simulink model "encoder2"  (R2022a)
settings: Solver=VariableStepAuto  StartTime=0.0  StopTime=10.0  RelTol=1e-3
libraries: simulink x3, spsSampleandHoldLib x1
settings Model: Creator=mluser  LastModifiedBy=mluser
settings ModelReferenceCC: EnableRefExpFcnMdlSchedulingChecks=off
settings RTWCC: Description=Generic Real-Time Target

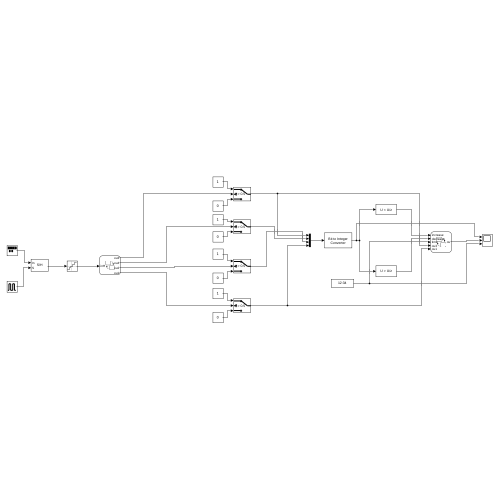
[thumbnail: Simulink's stored preview of the top-level diagram]
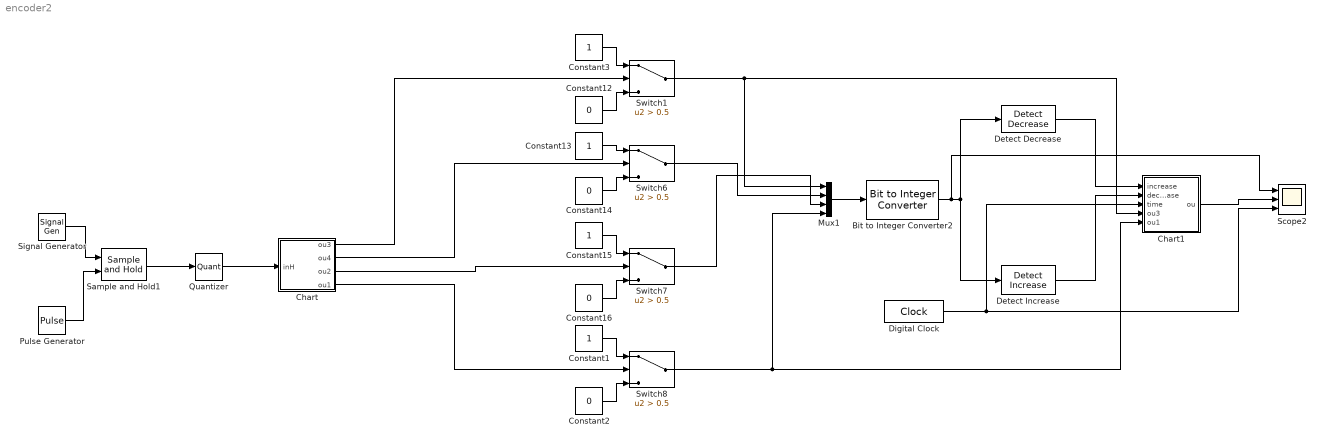
== system encoder2 ==
  Bit to Integer Converter2 : simulink/Logic and Bit Operations/Bit to Integer Converter  nbits=4  bitOrder=MSB first  signedOutputValues=Unsigned  outDtype=Inherit via internal rule  outDtypeSigned=Inherit via internal rule
  Chart : Stateflow chart  TreatAsAtomicUnit=on
  Chart1 : Stateflow chart  TreatAsAtomicUnit=on
  Constant{1,3,13,15} (4 alike) : Constant
  Constant{2,12,14,16} (4 alike) : Constant  Value=0
  Detect Decrease : simulink/Logic and Bit Operations/Detect Decrease  vinit=0.0  OutDataTypeStr=boolean
  Detect Increase : simulink/Logic and Bit Operations/Detect Increase  vinit=0.0  OutDataTypeStr=boolean
  Digital Clock : DigitalClock  SampleTime=0.1
  Mux1 : Mux
  Pulse Generator : DiscretePulseGenerator  PulseType=Time based  Period=0.1  PulseWidth=5
  Quantizer : Quantizer
  Sample and Hold1 : spsSampleandHoldLib/Sample and Hold  ic=0  Ts=0.1
  Scope2 : Scope  NumInputPorts=3
  Signal Generator : SignalGenerator  Amplitude=40  Units=rad/sec
  Switch{1,6..8} (4 alike) : Switch  Criteria=u2 > Threshold  Threshold=0.5  SaturateOnIntegerOverflow=off  InputSameDT=off
  wires:
  Pulse Generator/1 -> Sample and Hold1/2
  Signal Generator/1 -> Sample and Hold1/1
  Sample and Hold1/1 -> Quantizer/1
  Quantizer/1 -> Chart/1(inH)
  Constant3/1 -> Switch1/1
  Constant14/1 -> Switch6/3
  Chart/2(ou4) -> Switch6/2
  Switch7/1 -> Mux1/3
  Constant15/1 -> Switch7/1
  Constant13/1 -> Switch6/1
  Switch6/1 -> Mux1/2
  Chart/1(ou3) -> Switch1/2
  Constant16/1 -> Switch7/3
  Chart/3(ou2) -> Switch7/2
  Constant12/1 -> Switch1/3
  Switch1/1 -> Chart1/4(ou3), Mux1/1
  Constant1/1 -> Switch8/1
  Constant2/1 -> Switch8/3
  Chart/4(ou1) -> Switch8/2
  Switch8/1 -> Chart1/5(ou1), Mux1/4
  Mux1/1 -> Bit to Integer Converter2/1
  Bit to Integer Converter2/1 -> Scope2/1, Detect Decrease/1, Detect Increase/1
  Detect Decrease/1 -> Chart1/1(increase)
  Detect Increase/1 -> Chart1/2(decrease)
  Chart1/1(ou) -> Scope2/2
  Digital Clock/1 -> Scope2/3, Chart1/3(time)

== stateflow chart encoder2/Chart ==
  (default) -> (junction 3) : {ou1=0;
      | ou2=0;
      | ou3=0;
      | ou4=0;
      | }
  (junction 3) -> (junction 28) [order 2] : [inH==0]
  (junction 28) -> (junction 44) : {ou1=0;ou2=0;ou3=0;ou4=0;}
  (junction 3) -> (junction 10) [order 1]
  (junction 44) -> (junction 43)
  (junction 10) -> (junction 8) [order 1] : [inH<=10]
  (junction 8) -> (junction 43) : {ou1=1;ou2=0;ou3=0;ou4=0;}
  (junction 10) -> (junction 12) [order 2]
  (junction 43) -> (junction 42)
  (junction 16) -> (junction 42) : {ou1=1;ou2=1;ou3=0;ou4=0;}
  (junction 12) -> (junction 16) [order 1] : [inH>10&&inH<=20]
  (junction 42) -> (junction 41)
  (junction 12) -> (junction 19) [order 2]
  (junction 19) -> (junction 18) [order 1] : [inH>20&&inH<=30]
  (junction 18) -> (junction 41) : {ou1=1;ou2=1;ou3=1;ou4=0;}
  (junction 41) -> (junction 63)
  (junction 19) -> (junction 61) [order 2]
  (junction 61) -> (junction 62) : [inH>30]
  (junction 62) -> (junction 63) : {ou1=1;ou2=1;ou3=1;ou4=1;}
  data: ou3 output; ou4 output; ou2 output; ou1 output; inH input

== stateflow chart encoder2/Chart1 ==
  (default) -> (junction 3)
  (junction 3) -> (junction 28) [order 2] : [increase==1&&time>0]
  (junction 28) -> (junction 44) : {ou=1;}
  (junction 3) -> (junction 10) [order 1]
  (junction 44) -> (junction 43)
  (junction 10) -> (junction 8) [order 1] : [decrease==1&&time>0]
  (junction 8) -> (junction 43) : {ou=0;}
  (junction 10) -> (junction 71) [order 2]
  (junction 43) -> (junction 72)
  (junction 71) -> (junction 73) [order 1] : [time==0&&ou3==1]
  (junction 73) -> (junction 72) : {ou=1;}
  (junction 71) -> (junction 78) [order 2]
  (junction 72) -> (junction 80)
  (junction 78) -> (junction 79) : [time==0&&ou1==0]
  (junction 79) -> (junction 80) : {ou=0;}
  data: increase input; decrease input; ou output; time input; ou3 input; ou1 input
